simulink model "inverted_pendulum"  (R2018a)
settings: Solver=VariableStepAuto  StartTime=0.0  StopTime=inf  RelTol=1e-3
libraries: simulink x3
settings Model: Creator=RUPAM  LastModifiedBy=RUPAM

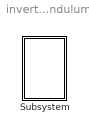
== system inverted_pendulum ==
  Subsystem : Subsystem

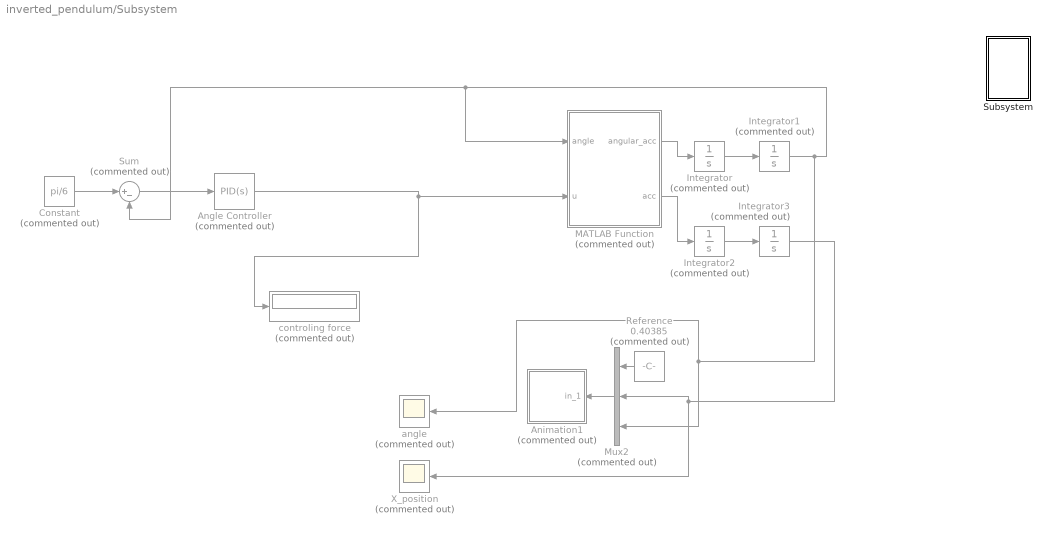
== system inverted_pendulum/Subsystem ==
  Angle Controller : simulink/Continuous/PID Controller  Commented=on  Controller=PID  TimeDomain=Continuous-time  SampleTime=-1  IntegratorMethod=Forward Euler  FilterMethod=Forward Euler  Form=Parallel  UseFilter=on  ControllerParametersSource=internal  P=-7691.26624395545  I=-26130.3354366134  D=-503.00427617919  N=66552.8826882912  InitialConditionSource=internal  InitialConditionForIntegrator=0  InitialConditionForFilter=0  ExternalReset=none  LimitOutput=off  UpperSaturationLimit=inf  LowerSaturationLimit=-inf  LinearizeAsGain=on  AntiWindupMode=none  Kb=1  TrackingMode=off  Kt=1  PParamMin=[]  PParamMax=[]  IParamMin=[]  IParamMax=[]  DParamMin=[]  DParamMax=[]  NParamMin=[]  NParamMax=[]  KbParamMin=[]  KbParamMax=[]  KtParamMin=[]  KtParamMax=[]  POutMin=[]  POutMax=[]  IOutMin=[]  IOutMax=[]  DOutMin=[]  DOutMax=[]  NOutMin=[]  NOutMax=[]  KbOutMin=[]  KbOutMax=[]  KtOutMin=[]  KtOutMax=[]  IntegratorOutMin=[]  IntegratorOutMax=[]  FilterOutMin=[]  FilterOutMax=[]  SumOutMin=[]  SumOutMax=[]  SumI1OutMin=[]  SumI1OutMax=[]  SumI2OutMin=[]  SumI2OutMax=[]  SumI3OutMin=[]  SumI3OutMax=[]  SumDOutMin=[]  SumDOutMax=[]  SaturationOutMin=[]  SaturationOutMax=[]  IntegratorContinuousStateAttributes=''  IntegratorStateMustResolveToSignalObject=off  IntegratorRTWStateStorageClass=Auto  FilterContinuousStateAttributes=''  FilterStateMustResolveToSignalObject=off  FilterRTWStateStorageClass=Auto  DifferentiatorICPrevScaledInput=0  DifferentiatorOutMin=[]  DifferentiatorOutMax=[]  FilterDiffOutCoefMin=[]  FilterDiffOutCoefMax=[]  SumDenOutMin=[]  SumDenOutMax=[]  SumNumOutMin=[]  SumNumOutMax=[]  ReciprocalOutMin=[]  ReciprocalOutMax=[]  DivideOutMin=[]  DivideOutMax=[]  TunerSelectOption=Transfer Function Based (PID Tuner App)
  Animation1 : Subsystem  Commented=on  mask(Pendulum plot){RefBlock=Reference, Parameter2=0}
      mask prompts: RefBlock "DC reference signal block name:"
      mask help: Pendulum plot
      mask Help: Pendulum animation function using Handle graphics.
      mask Display: plot([-100 100],[0 0],[-2 -2 2 2],[0 1 1 0],[0 3],[1 5])
  Constant : Constant  Commented=on  Value=pi/6
  Integrator{,1..3} (4 alike) : Integrator  Commented=on
  MATLAB Function : MATLAB Function  Commented=on  TreatAsAtomicUnit=on
  Mux2 : Mux  Commented=on  Inputs=3
  Reference : Constant  Commented=on  Value=0.40385
  Subsystem : Subsystem
  Sum : Sum  Commented=on  Inputs=|+-
  X_position : Scope  Commented=on
  angle : Scope  Commented=on
  controling force : Display  Commented=on
  wires:
  Integrator1/1 -> Mux2/3, angle/1, MATLAB Function/1(angle), Sum/2
  Integrator3/1 -> Mux2/2, X_position/1
  Integrator/1 -> Integrator1/1
  Mux2/1 -> Animation1/1(in_1)
  MATLAB Function/2(acc) -> Integrator2/1
  MATLAB Function/1(angular_acc) -> Integrator/1
  Sum/1 -> Angle Controller/1
  Integrator2/1 -> Integrator3/1
  Angle Controller/1 -> MATLAB Function/2(u), controling force/1
  Constant/1 -> Sum/1
  Reference/1 -> Mux2/1

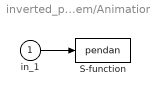
== system inverted_pendulum/Subsystem/Animation1 ==
  in_1 : Inport
  S-function : S-Function  FunctionName=pendan  Parameters=RefBlock  SFunctionDeploymentMode=off  EnableBusSupport=off
      settings: DeleteFcn=pendan([],[],[],'DeleteBlock');
  wires:
  in_1/1 -> S-function/1

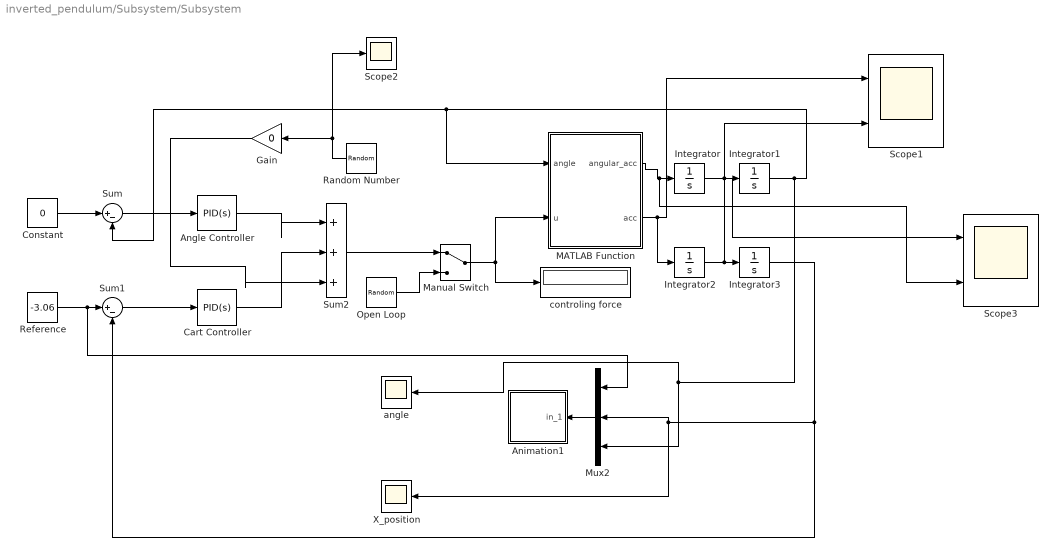
== system inverted_pendulum/Subsystem/Subsystem ==
  Angle Controller : simulink/Continuous/PID Controller  Controller=PID  TimeDomain=Continuous-time  SampleTime=-1  IntegratorMethod=Forward Euler  FilterMethod=Forward Euler  Form=Parallel  UseFilter=on  ControllerParametersSource=internal  P=-7691.26624395545  I=-26130.3354366134  D=-600.00427617919  N=66552.8826882912  InitialConditionSource=internal  InitialConditionForIntegrator=0  InitialConditionForFilter=0  ExternalReset=none  LimitOutput=off  UpperSaturationLimit=inf  LowerSaturationLimit=-inf  LinearizeAsGain=on  AntiWindupMode=none  Kb=1  TrackingMode=off  Kt=1  PParamMin=[]  PParamMax=[]  IParamMin=[]  IParamMax=[]  DParamMin=[]  DParamMax=[]  NParamMin=[]  NParamMax=[]  KbParamMin=[]  KbParamMax=[]  KtParamMin=[]  KtParamMax=[]  POutMin=[]  POutMax=[]  IOutMin=[]  IOutMax=[]  DOutMin=[]  DOutMax=[]  NOutMin=[]  NOutMax=[]  KbOutMin=[]  KbOutMax=[]  KtOutMin=[]  KtOutMax=[]  IntegratorOutMin=[]  IntegratorOutMax=[]  FilterOutMin=[]  FilterOutMax=[]  SumOutMin=[]  SumOutMax=[]  SumI1OutMin=[]  SumI1OutMax=[]  SumI2OutMin=[]  SumI2OutMax=[]  SumI3OutMin=[]  SumI3OutMax=[]  SumDOutMin=[]  SumDOutMax=[]  SaturationOutMin=[]  SaturationOutMax=[]  IntegratorContinuousStateAttributes=''  IntegratorStateMustResolveToSignalObject=off  IntegratorRTWStateStorageClass=Auto  FilterContinuousStateAttributes=''  FilterStateMustResolveToSignalObject=off  FilterRTWStateStorageClass=Auto  DifferentiatorICPrevScaledInput=0  DifferentiatorOutMin=[]  DifferentiatorOutMax=[]  FilterDiffOutCoefMin=[]  FilterDiffOutCoefMax=[]  SumDenOutMin=[]  SumDenOutMax=[]  SumNumOutMin=[]  SumNumOutMax=[]  ReciprocalOutMin=[]  ReciprocalOutMax=[]  DivideOutMin=[]  DivideOutMax=[]  TunerSelectOption=Transfer Function Based (PID Tuner App)
  Animation1 : Subsystem  mask(Pendulum plot){RefBlock=Reference, Parameter2=0}
      mask prompts: RefBlock "DC reference signal block name:"
      mask help: Pendulum plot
      mask Help: Pendulum animation function using Handle graphics.
      mask Display: plot([-100 100],[0 0],[-2 -2 2 2],[0 1 1 0],[0 3],[1 5])
  Cart Controller : simulink/Continuous/PID Controller  Controller=PID  TimeDomain=Continuous-time  SampleTime=-1  IntegratorMethod=Forward Euler  FilterMethod=Forward Euler  Form=Parallel  UseFilter=on  ControllerParametersSource=internal  P=-3240.3861619702  I=-787.146927150774  D=-587.45153333948  N=1.40524226520522  InitialConditionSource=internal  InitialConditionForIntegrator=0  InitialConditionForFilter=0  ExternalReset=none  LimitOutput=off  UpperSaturationLimit=inf  LowerSaturationLimit=-inf  LinearizeAsGain=on  AntiWindupMode=none  Kb=1  TrackingMode=off  Kt=1  PParamMin=[]  PParamMax=[]  IParamMin=[]  IParamMax=[]  DParamMin=[]  DParamMax=[]  NParamMin=[]  NParamMax=[]  KbParamMin=[]  KbParamMax=[]  KtParamMin=[]  KtParamMax=[]  POutMin=[]  POutMax=[]  IOutMin=[]  IOutMax=[]  DOutMin=[]  DOutMax=[]  NOutMin=[]  NOutMax=[]  KbOutMin=[]  KbOutMax=[]  KtOutMin=[]  KtOutMax=[]  IntegratorOutMin=[]  IntegratorOutMax=[]  FilterOutMin=[]  FilterOutMax=[]  SumOutMin=[]  SumOutMax=[]  SumI1OutMin=[]  SumI1OutMax=[]  SumI2OutMin=[]  SumI2OutMax=[]  SumI3OutMin=[]  SumI3OutMax=[]  SumDOutMin=[]  SumDOutMax=[]  SaturationOutMin=[]  SaturationOutMax=[]  IntegratorContinuousStateAttributes=''  IntegratorStateMustResolveToSignalObject=off  IntegratorRTWStateStorageClass=Auto  FilterContinuousStateAttributes=''  FilterStateMustResolveToSignalObject=off  FilterRTWStateStorageClass=Auto  DifferentiatorICPrevScaledInput=0  DifferentiatorOutMin=[]  DifferentiatorOutMax=[]  FilterDiffOutCoefMin=[]  FilterDiffOutCoefMax=[]  SumDenOutMin=[]  SumDenOutMax=[]  SumNumOutMin=[]  SumNumOutMax=[]  ReciprocalOutMin=[]  ReciprocalOutMax=[]  DivideOutMin=[]  DivideOutMax=[]  TunerSelectOption=Transfer Function Based (PID Tuner App)
  Constant : Constant  Value=0
  Gain : Gain  Gain=0
  Integrator{,1..3} (4 alike) : Integrator
  MATLAB Function : MATLAB Function  TreatAsAtomicUnit=on
  Manual Switch : ManualSwitch
  Mux2 : Mux  Inputs=3
  Open Loop : RandomNumber  SampleTime=0.1
  Random Number : RandomNumber  SampleTime=0.1
  Reference : Constant  Value=-3.06
  Scope1 : Scope  NumInputPorts=2
  Scope2 : Scope
  Scope3 : Scope  NumInputPorts=2
  Sum : Sum  Inputs=|+-
  Sum1 : Sum  Inputs=|+-
  Sum2 : Sum  Inputs=|+++
  X_position : Scope
  angle : Scope
  controling force : Display
  wires:
  MATLAB Function/1(angular_acc) -> Scope3/2, Integrator/1
  Constant/1 -> Sum/1
  Gain/1 -> Sum2/3
  Integrator3/1 -> Mux2/2, X_position/1, Sum1/2
  Manual Switch/1 -> controling force/1, MATLAB Function/2(u)
  Cart Controller/1 -> Sum2/2
  Integrator1/1 -> Mux2/3, angle/1, MATLAB Function/1(angle), Sum/2
  Integrator2/1 -> Scope1/2, Integrator3/1
  Sum/1 -> Angle Controller/1
  Open Loop/1 -> Manual Switch/2
  Sum1/1 -> Cart Controller/1
  Reference/1 -> Mux2/1, Sum1/1
  MATLAB Function/2(acc) -> Scope1/1, Integrator2/1
  Integrator/1 -> Scope3/1, Integrator1/1
  Mux2/1 -> Animation1/1(in_1)
  Angle Controller/1 -> Sum2/1
  Random Number/1 -> Gain/1, Scope2/1
  Sum2/1 -> Manual Switch/1

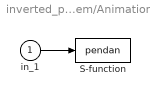
== system inverted_pendulum/Subsystem/Subsystem/Animation1 ==
  in_1 : Inport
  S-function : S-Function  FunctionName=pendan  Parameters=RefBlock  SFunctionDeploymentMode=off  EnableBusSupport=off
      settings: DeleteFcn=pendan([],[],[],'DeleteBlock');
  wires:
  in_1/1 -> S-function/1

== matlab function inverted_pendulum/Subsystem/MATLAB Function ==
  data: angle input; u input; angular_acc output; acc output
function [angular_acc,acc] = fcn(angle,u)
M=2.4;
m=0.23;
l=0.36;
g=9.8;

angular_acc=(((M+m)*g*angle)-(u))/(M*l);

acc=(u-(m*g*angle))/M;

== matlab function inverted_pendulum/Subsystem/Subsystem/MATLAB Function ==
  data: angle input; u input; angular_acc output; acc output
function [angular_acc,acc] = fcn(angle,u)
M=2.4;
m=0.23;
l=0.36;
g=9.8;

angular_acc=(((M+m)*g*angle)-(u))/(M*l);

acc=(u-(m*g*angle))/M;
